simulink model "lab0_1"  (R2021a)
settings: Solver=VariableStepAuto  StartTime=0.0  StopTime=0.05  RelTol=1e-3
settings Model: Creator=Giancarlo  LastModifiedBy=Giancarlo

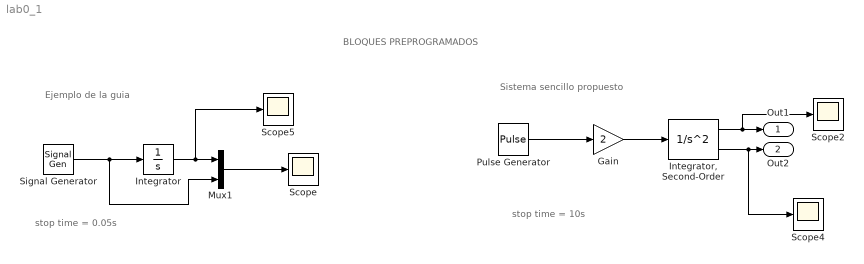
== system lab0_1 ==
  note: stop time = 10s
  note: stop time = 0.05s
  note: BLOQUES PREPROGRAMADOS
  note: Sistema sencillo propuesto
  note: Ejemplo de la guia
  Gain : Gain  Gain=2
  Integrator : Integrator
  "Integrator, Second-Order" : SecondOrderIntegrator
  Mux1 : Mux  Inputs=2
  Pulse Generator : DiscretePulseGenerator  PulseType=Time based  Period=10  PulseWidth=5
  Scope{,2,4..5} (4 alike) : Scope
  Signal Generator : SignalGenerator  Amplitude=10  Frequency=60
  Out1 : Outport
  Out2 : Outport  Port=2
  wires:
  Signal Generator/1 -> Mux1/2, Integrator/1
  Integrator/1 -> Mux1/1, Scope5/1
  Mux1/1 -> Scope/1
  Pulse Generator/1 -> Gain/1
  Gain/1 -> "Integrator, Second-Order"/1
  "Integrator, Second-Order"/1 -> Out1/1, Scope2/1
  "Integrator, Second-Order"/2 -> Scope4/1, Out2/1
